simulink model "BPSK"  (R2023b)
settings: Solver=VariableStepAuto  StartTime=0.0  StopTime=10  RelTol=1e-3
libraries: commrandsrc3 x1, commrflib2 x1
settings Model: Creator=HP  LastModifiedBy=HP

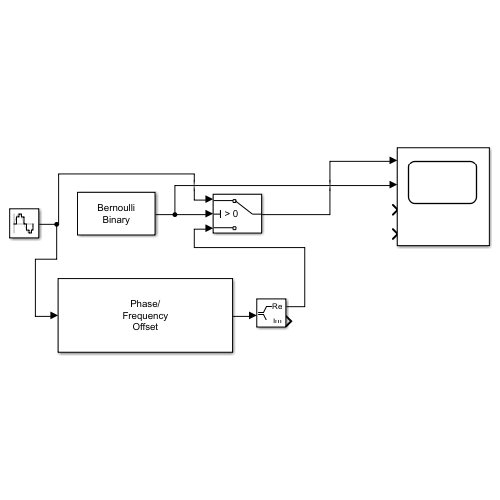
[thumbnail: Simulink's stored preview of the top-level diagram]
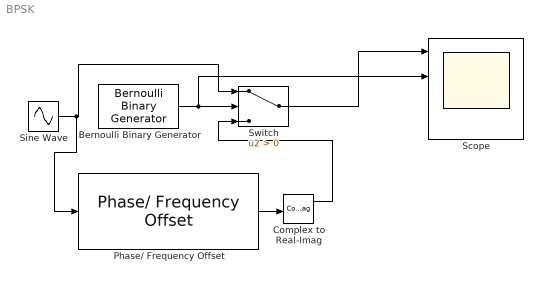
== system BPSK ==
  Bernoulli Binary Generator : commrandsrc3/Bernoulli Binary Generator  ProbabilityOfZero=0.5  SeedSource=Auto  Seed=0  SampleTime=1  SamplesPerFrame=1  OutputDataType=double  SimulateUsing=Interpreted execution
  Complex to Real-Imag : ComplexToRealImag
  Phase/ Frequency Offset : commrflib2/Phase// Frequency Offset  phaseOffset=180  freqPort=off  freqOffset=0
      settings: LibrarySourceBlock=|
      | commrfcorlib/Phase//
      | Frequency
      | Offset
  Scope : Scope  NumInputPorts=4
  Sine Wave : Sin  Frequency=2*pi  SampleTime=0.01
  Switch : Switch  Criteria=u2 > Threshold  SaturateOnIntegerOverflow=off  InputSameDT=off
  wires:
  Bernoulli Binary Generator/1 -> Scope/2, Switch/2
  Switch/1 -> Scope/1
  Sine Wave/1 -> Phase/ Frequency Offset/1, Switch/1
  Phase/ Frequency Offset/1 -> Complex to Real-Imag/1
  Complex to Real-Imag/1 -> Switch/3
